simulink model "prueva"  (R2015b)
settings: Solver=VariableStepAuto  StartTime=0.0  StopTime=5  RelTol=1e-3
settings Model: Creator=nikol  LastModifiedBy=nikol

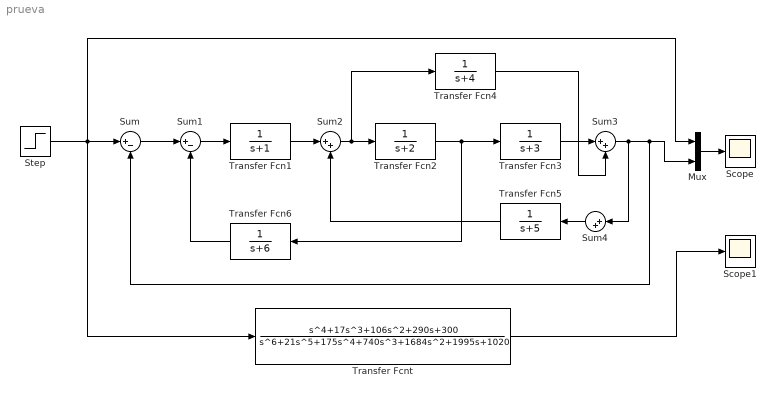
== system prueva ==
  Mux : Mux  Inputs=2
  Scope : Scope
  Scope1 : Scope
  Step : Step  SampleTime=0
  Sum : Sum  Inputs=|+-
  Sum1 : Sum  Inputs=|+-
  Sum2 : Sum  Inputs=|++
  Sum3 : Sum  Inputs=|++
  Sum4 : Sum  Inputs=|++
  Transfer Fcn1 : TransferFcn  Denominator=[1 1]
  Transfer Fcn2 : TransferFcn  Denominator=[1 2]
  Transfer Fcn3 : TransferFcn  Denominator=[1 3]
  Transfer Fcn4 : TransferFcn  Denominator=[1 4]
  Transfer Fcn5 : TransferFcn  Denominator=[1 5]
  Transfer Fcn6 : TransferFcn  Denominator=[1 6]
  Transfer Fcnt : TransferFcn  Numerator=[1 17 106 290 300]  Denominator=[1 21 175 740 1684 1995 1020]
  wires:
  Mux/1 -> Scope/1
  Step/1 -> Mux/1, Transfer Fcnt/1, Sum/1
  Sum/1 -> Sum1/1
  Sum1/1 -> Transfer Fcn1/1
  Transfer Fcn1/1 -> Sum2/1
  Sum2/1 -> Transfer Fcn4/1, Transfer Fcn2/1
  Transfer Fcn2/1 -> Transfer Fcn6/1, Transfer Fcn3/1
  Transfer Fcn3/1 -> Sum3/1
  Transfer Fcn4/1 -> Sum3/2
  Transfer Fcn5/1 -> Sum2/2
  Transfer Fcn6/1 -> Sum1/2
  Sum3/1 -> Sum4/1, Mux/2, Sum/2
  Sum4/1 -> Transfer Fcn5/1
  Transfer Fcnt/1 -> Scope1/1
